simulink model "Modelo_control_d_2GDL_2021"  (R2021b)
settings: Solver=ode45  StartTime=0.0  StopTime=20  MaxStep=1e-5  RelTol=1e-9
undefined symbols (not defined in the file or in its folder): airgap, current_I, currentSensorNoise, DiscIntNeverNeededParam, dtCurrent, dTSensor, filterConstant, inductance, initial_conds, K_d, Ki, Kp, noiseSensor, pod, Rcoil, resCurrent, T, tauFilterCurrent, thetafilter, z_0, z_ini, z_lev
libraries: cstblocks x5, slpidlib x3, simulink_extras x1
(part 2 of 2)

== matlab function Modelo_control_d_2GDL_2021/Modelo no-lineal/Non-linear 3 DOF model/H7 Pod Dynamic model (3DOF)/Levitation /MATLAB Function1 ==
  data: airgap input; F output; intensity input; pod parameter
function F = HEMSlev(airgap, intensity, pod)
% Computes the levitation force (N) of all the HEMS units as a function of 
% their air gaps (mm) and intensities (A)
% ═════════════════════════════════════════════════════════════════════════
% Last updated: 15.12.2021
% ════════════════════════════════════════════════════════════════════════

x   = airgap;
y   = intensity;

F = pod.levitation.poly_1_unit.p00 + ...
    pod.levitation.poly_1_unit.p10.*x + ...
    pod.levitation.poly_1_unit.p01.*y + ...
    pod.levitation.poly_1_unit.p20.*x.^2 + ...
    pod.levitation.poly_1_unit.p11.*x.*y + ...
    pod.levitation.poly_1_unit.p02.*y.^2 + ...
    pod.levitation.poly_1_unit.p21.*x.^2.*y + ...
    pod.levitation.poly_1_unit.p12.*x.*y.^2 + ...
    pod.levitation.poly_1_unit.p03.*y.^3;

== matlab function Modelo_control_d_2GDL_2021/Modelo no-lineal/Non-linear 3 DOF model/H7 Pod Dynamic model (3DOF)/Wheels /MATLAB Function ==
  data: F output; pod parameter; z_CF output
function [F, z_CF] = rollingFriction(pod)
% Computes the rolling resistance force (N) of the wheels. It distinguishes
% 3 cases: 
%   (1) z = 0. Pod touching the ground
%   (2) z = z_max. Pod touching the ceiling. It is assumed no current
%   applied to the HEMS. 
%   (3) Otherwise. Pod levitating. 
% ═════════════════════════════════════════════════════════════════════════
% Last updated: 26.12.2021
% ═════════════════════════════════════════════════════════════════════════

% F_LEV worst case scenario computation
% x   = 12; % [mm]
% y   = 0;  % [A]
% 
% F_LEV = pod.levitation.poly_1_unit.p00 + ...
%         pod.levitation.poly_1_unit.p10.*x + ...
%         pod.levitation.poly_1_unit.p01.*y + ...
%         pod.levitation.poly_1_unit.p20.*x.^2 + ...
%         pod.levitation.poly_1_unit.p11.*x.*y + ...
%         pod.levitation.poly_1_unit.p02.*y.^2 + ...
%         pod.levitation.poly_1_unit.p21.*x.^2.*y + ...
%         pod.levitation.poly_1_unit.p12.*x.*y.^2 + ...
%         pod.levitation.poly_1_unit.p03.*y.^3;

% % Main algorithm
% if z == 0
%     F_N   = pod.mass.mass * 9.81;
%     z_CF  = - pod.geometry.z_CF;
% elseif z == pod.general.z_range
%     F_N   = 6 * F_LEV - pod.mass.mass * 9.81;
%     z_CF  = pod.geometry.z_CF;
% else
%     F_N   = 0;
%     z_CF  = 0;
% end

F_N    = pod.mass.mass * 9.81;
z_CF  = - pod.geometry.z_CF;

F = pod.wheels.number * pod.wheels.roll_coef * F_N;
